simulink model "sim_control_two_DOF_robot_manipulator"  (R2023a)
settings: Solver=VariableStepAuto  StartTime=0.0  StopTime=3  RelTol=1e-3
settings Model: Creator=ACCENT  LastModifiedBy=ACCENT

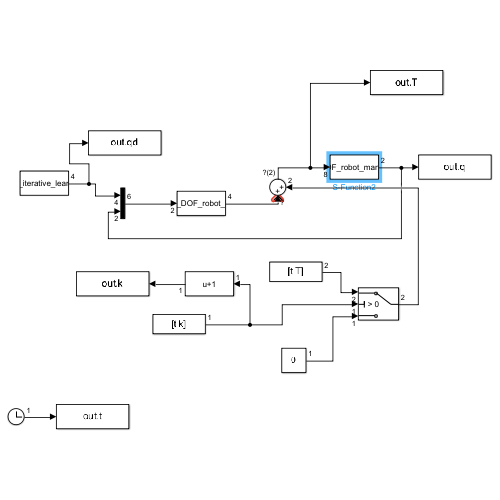
[thumbnail: Simulink's stored preview of the top-level diagram]
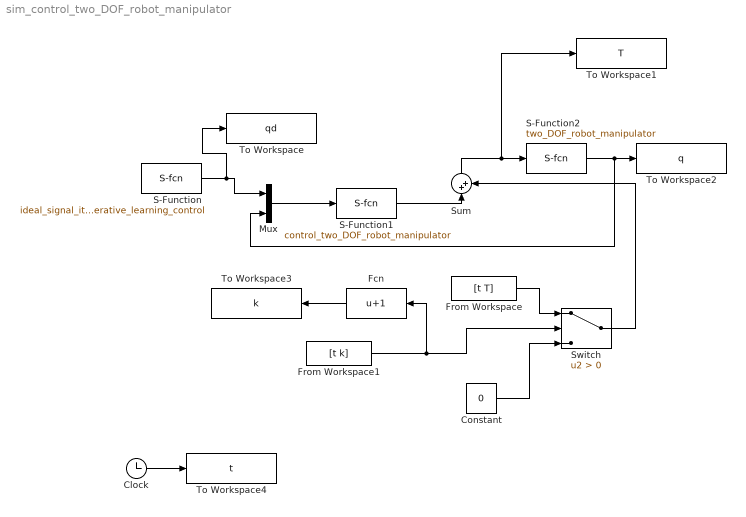
== system sim_control_two_DOF_robot_manipulator ==
  Clock : Clock
      settings: Decimation=3
  Constant : Constant  Value=0
  Fcn : Fcn  Expr=u+1
  From Workspace : FromWorkspace  VariableName=[t T]
  From Workspace1 : FromWorkspace  VariableName=[t k]
  Mux : Mux  Inputs=2
  S-Function : S-Function  FunctionName=ideal_signal_iterative_learning_control  SFunctionDeploymentMode=off  EnableBusSupport=off
  S-Function1 : S-Function  FunctionName=control_two_DOF_robot_manipulator  SFunctionDeploymentMode=off  EnableBusSupport=off
  S-Function2 : S-Function  FunctionName=two_DOF_robot_manipulator  SFunctionDeploymentMode=off  EnableBusSupport=off
  Sum : Sum  Inputs=|++
  Switch : Switch  Criteria=u2 > Threshold  SaturateOnIntegerOverflow=off  InputSameDT=off
  To Workspace : ToWorkspace  VariableName=qd  SampleTime=-1
  To Workspace1 : ToWorkspace  VariableName=T  SampleTime=-1
  To Workspace2 : ToWorkspace  VariableName=q  SampleTime=-1
  To Workspace3 : ToWorkspace  VariableName=k  SampleTime=-1
  To Workspace4 : ToWorkspace  VariableName=t  SampleTime=-1
  wires:
  Clock/1 -> To Workspace4/1
  Fcn/1 -> To Workspace3/1
  From Workspace1/1 -> Fcn/1, Switch/2
  From Workspace/1 -> Switch/1
  Constant/1 -> Switch/3
  Switch/1 -> Sum/2
  S-Function/1 -> To Workspace/1, Mux/1
  Mux/1 -> S-Function1/1
  S-Function1/1 -> Sum/1
  Sum/1 -> To Workspace1/1, S-Function2/1
  S-Function2/1 -> Mux/2, To Workspace2/1
